simulink model "RC_Servo_Model"  (R2022a)
settings: Solver=VariableStepAuto  StartTime=0.0  StopTime=1  FixedStep=0.001  RelTol=1e-3
undefined symbols (not defined in the file): B, FoV_w, J, K_tau, K_v, La, Pixel_w, Ra
libraries: fl_lib x4, nesl_utility x3, ee_lib x3, simulink_extras x2, simulink x1, slpidlib x1
settings Model: Creator=bobjo  LastModifiedBy=bobjo
settings SolverCC: EnableFixedStepZeroCrossing=on

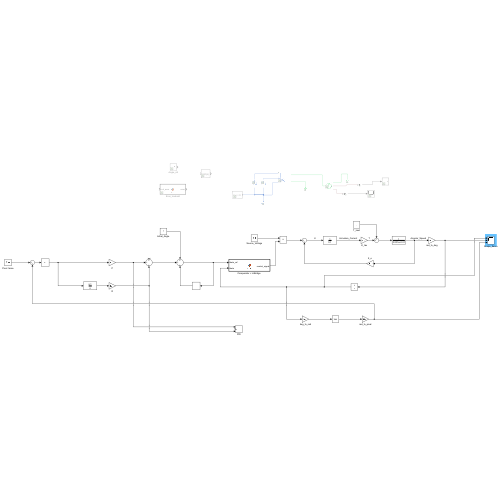
[thumbnail: Simulink's stored preview of the top-level diagram]
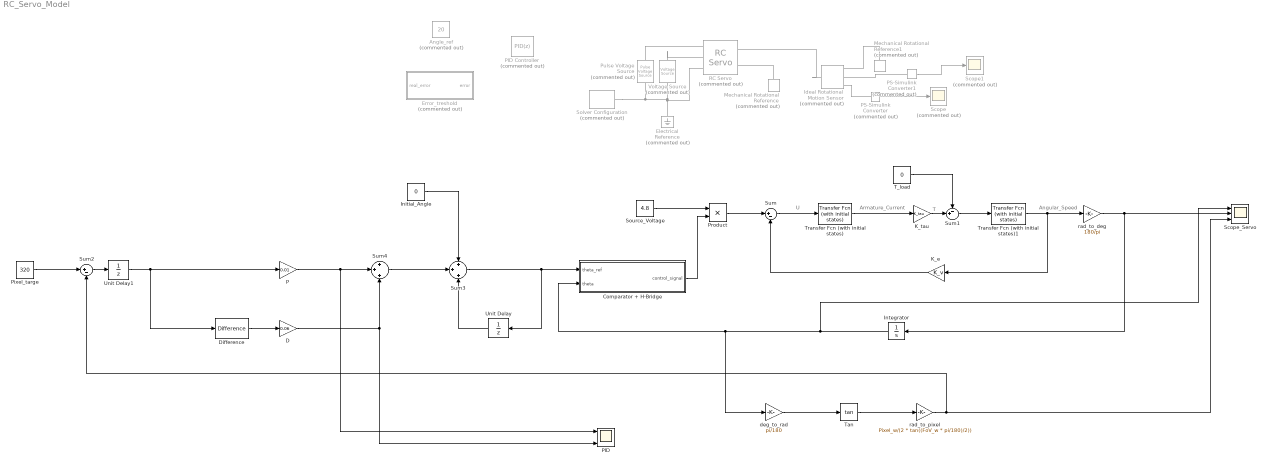
== system RC_Servo_Model ==
  note: Armature_Current
  note: Angular_Speed
  note: T
  note: U
  Angle_ref : Constant  Commented=on  Value=20
  "Comparator + H-Bridge " : MATLAB Function  TreatAsAtomicUnit=on
  D : Gain  Gain=0.06
  Difference : simulink/Discrete/Difference  ICPrevInput=0.0  OutMin=[]  OutMax=[]  OutDataType=fixdt(1, 16)  OutScaling=2^-10  DoSatur=off
  Electrical Reference : fl_lib/Electrical/Electrical Elements/Electrical Reference  Commented=on
      settings: SourceProductBaseCode=PW,SS,VE
  Error_treshold : MATLAB Function  Commented=on  TreatAsAtomicUnit=on
  Ideal Rotational Motion Sensor : fl_lib/Mechanical/Mechanical Sensors/Ideal Rotational Motion Sensor  Commented=on  wrap_angle=simscape.enum.onoff.off  offset=0 rad
      settings: SourceProductBaseCode=PW,SS,VE
  Initial_Angle : Constant  Value=0
  Integrator : Integrator
  K_e : Gain  Gain=K_v
  K_tau : Gain  Gain=K_tau
  Mechanical Rotational Reference : fl_lib/Mechanical/Rotational Elements/Mechanical Rotational Reference  Commented=on
      settings: SourceProductBaseCode=PW,SS,VE
  Mechanical Rotational Reference1 : fl_lib/Mechanical/Rotational Elements/Mechanical Rotational Reference  Commented=on
      settings: SourceProductBaseCode=PW,SS,VE
  P : Gain  Gain=0.01
  PID : Scope  NumInputPorts=3
  PID Controller : slpidlib/PID Controller  Commented=on  Controller=PID  Form=Parallel  TimeDomain=Discrete-time  UseExternalTs=off  SampleTime=0.01  IntegratorMethod=Forward Euler  FilterMethod=Forward Euler  ControllerParametersSource=internal  P=0  I=0  UseKiTs=off  D=0.2 * 0.01  N=100  UseFilter=on  TunerSelectOption=Transfer Function Based (PID Tuner App)  InitialConditionSource=internal  InitialConditionForIntegrator=0  InitialConditionForFilter=0  DifferentiatorICPrevScaledInput=0  ExternalReset=none  TrackingMode=off  Kt=1  LimitOutput=off  SatLimitsSource=internal  UpperSaturationLimit=inf  LowerSaturationLimit=-inf  LinearizeAsGain=on  AntiWindupMode=none  Kb=1  POutMin=[]  POutMax=[]  IOutMin=[]  IOutMax=[]  DOutMin=[]  DOutMax=[]  NOutMin=[]  NOutMax=[]  SumOutMin=[]  SumOutMax=[]  SaturationOutMin=[]  SaturationOutMax=[]  PParamMin=[]  PParamMax=[]  IParamMin=[]  IParamMax=[]  DParamMin=[]  DParamMax=[]  NParamMin=[]  NParamMax=[]  KbParamMin=[]  KbParamMax=[]  KtParamMin=[]  KtParamMax=[]  KbOutMin=[]  KbOutMax=[]  KtOutMin=[]  KtOutMax=[]  IntegratorOutMin=[]  IntegratorOutMax=[]  FilterOutMin=[]  FilterOutMax=[]  SumI1OutMin=[]  SumI1OutMax=[]  SumI2OutMin=[]  SumI2OutMax=[]  SumI3OutMin=[]  SumI3OutMax=[]  SumI4OutMin=[]  SumI4OutMax=[]  SumDOutMin=[]  SumDOutMax=[]  DifferentiatorOutMin=[]  DifferentiatorOutMax=[]  FilterDiffOutCoefMin=[]  FilterDiffOutCoefMax=[]  ReciprocalOutMin=[]  ReciprocalOutMax=[]  SumDenOutMin=[]  SumDenOutMax=[]  SumNumOutMin=[]  SumNumOutMax=[]  DivideOutMin=[]  DivideOutMax=[]  UdiffTsProdOutMin=[]  UdiffTsProdOutMax=[]  NTsProdOutMin=[]  NTsProdOutMax=[]  UintegralTsProdOutMin=[]  UintegralTsProdOutMax=[]  UngainTsProdOutMin=[]  UngainTsProdOutMax=[]  IntegratorContinuousStateAttributes=''  IntegratorStateMustResolveToSignalObject=off  IntegratorRTWStateStorageClass=Auto  FilterContinuousStateAttributes=''  FilterStateMustResolveToSignalObject=off  FilterRTWStateStorageClass=Auto  ParallelPVariant=InternalParameters  IdealPVariant=Disabled  IVariant=InternalParameters  DVariant=InternalParameters  IntegratorVariant=Discrete  SatVariant=Disabled  AWVariant=Passthrough  PCopyVariant=Disabled  TRVariant=Disabled  FdbkBlocksVariant=Forward  IdealPFdbkVariant=Disabled  SatFdbkVariant=Disabled  DerivativeFilterVariant=ForwardEulerFilter  NVariant=InternalParameters  NCopyVariant=Disabled  FilterICVariant=InternalICsFilter  IntegratorICVariant=InternalICs  ExternalResetVariant=Disabled  TRSumVariant=Passthrough  SumFdbkVariant=Disabled  SumVariant=Sum_PID  TsampFilterVariant=InternalTs  TsampNgainVariant=Passthrough  TsampIntegralVariant=Passthrough  ExternalSaturationOutDataTypeStr=Inherit: Same as second input  aMode=0
  PS-Simulink Converter : nesl_utility/PS-Simulink Converter  Commented=on  PhysicalDomain=network_engine_domain  SubClassName=ps_output  LeftPortType=input  RightPortType=output  PseudoPeriodic=off  Frequencies=[]  VectorFormat=inherit  Unit=deg  AffineConversion=off
      settings: SourceProductBaseCode=SS,PW,VE
  PS-Simulink Converter1 : nesl_utility/PS-Simulink Converter  Commented=on  PhysicalDomain=network_engine_domain  SubClassName=ps_output  LeftPortType=input  RightPortType=output  PseudoPeriodic=off  Frequencies=[]  VectorFormat=inherit  Unit=deg/s  AffineConversion=off
      settings: SourceProductBaseCode=SS,PW,VE
  Pixel_targe : Constant  Value=320
  Product : Product
  Pulse Voltage Source : ee_lib/Additional Components/SPICE Sources/Pulse Voltage Source  Commented=on  V1=0 V  V2=5 V  TD=0.1 s  TR=1e-9 s  TF=1e-9 s  PW=0.5 ms  PER=20 ms
      settings: SourceProductBaseCode=PS  InternalSimscapePortConfiguration="{\"Bottom\":[],\"Left\":[{\"id\":\"p\",\"label\":\"\",\"type\":\"foundation.electrical.electrical\"}],\"Right\":[{\"id\":\"n\",\"label\":\"\",\"type\":\"foundation.electrical.electrical\"}],\"Top\":[]}"
  RC Servo : ee_lib/Electromechanical/Brushed Motors/RC Servo  Commented=on  stall_torque=1.8 cm*kg  time_60=0.2 s  nominal_voltage=5 V  rotational_range=[0, 180] deg  pulse_width_range=[500, 2500] us  threshold=3 V  R_s=18 kOhm  resolution=1 deg  angle_meas_error=0 deg  backdrive_torque=0.5 cm*kg  ratio=320  inertia=0.01 cm^2*g  endstop_angles=[-5, 185] deg  endstop_stiffness=1e6 N*m/rad  endstop_damping=0.01 N*m*s/rad  enable_faults=0  fault_action=1  fault_type=1  enable_temporal_fault=0  t_fault=1 s  enable_behavioral_fault=0  max_permissible_current=1 A  t_fail_on_current=1 s  angle_specify=off  angle_priority=High  angle=90 deg  angle_nominal_specify=off  angle_nominal_unit=deg  angle_nominal_value=1  w_specify=off  w_priority=High  w=0 deg/s  w_nominal_specify=off  w_nominal_unit=deg/s  w_nominal_value=1  torque_specify=off  torque_priority=None  torque=0 N*m  torque_nominal_specify=off  torque_nominal_unit=N*m  torque_nominal_value=1  pulse_width_specify=off  pulse_width_priority=Low  pulse_width=1.5 ms  i_specify=off  i_priority=None  i=0 A  i_nominal_specify=off  i_nominal_unit=A  i_nominal_value=1  i_s_specify=off  i_s_priority=None  i_s=0 A  i_s_nominal_specify=off  i_s_nominal_unit=A  i_s_nominal_value=1  motor_torque_specify=off  motor_torque_priority=None  motor_torque=0 N*m  motor_torque_nominal_specify=off  motor_torque_nominal_unit=N*m  motor_torque_nominal_value=1  power_dissipated_specify=off  power_dissipated_priority=None  power_dissipated=0 W  power_dissipated_nominal_specify=off  power_dissipated_nominal_unit=W  power_dissipated_nominal_value=1  angle_demand_specify=off  angle_demand_priority=None  angle_demand=90 deg  angle_demand_nominal_specify=off  angle_demand_nominal_unit=deg  angle_demand_nominal_value=1  faulted_specify=off  faulted_priority=None  faulted=0  faulted_nominal_specify=off  faulted_nominal_unit=1  faulted_nominal_value=1
      settings: SourceProductBaseCode=PS  InternalSimscapePortConfiguration="{\"Bottom\":[],\"Left\":[{\"id\":\"s\",\"label\":\"s\",\"type\":\"foundation.electrical.electrical\"},{\"id\":\"p\",\"label\":\"+\",\"type\":\"foundation.electrical.electrical\"},{\"id\":\"n\",\"label\":\"-\",\"type\":\"foundation.electrical.electrical\"}],\"Right\":[{\"id\":\"R\",\"label\":\"R\",\"type\":\"foundation.mechanical.rotational.rotational\"},{\"id\":\"C\",\"label\":\"C\",\"type\":\"foundation.mechanical.rotational.rotational\"}],\"Top\":[]}"
  Scope : Scope  Commented=on
  Scope1 : Scope  Commented=on
  Scope_Servo : Scope  NumInputPorts=3
  Solver Configuration : nesl_utility/Solver Configuration  Commented=on  PhysicalDomain=network_engine_domain  SubClassName=solver  LeftPortType=input  RightPortType=generic  Tones=[]  Harmonics=[]  SimulateNoise=off  Profile=off  UseLocalSampling=off  EnableSwitchedLinearOptims=on  FrequencyDomain=off  UseCCode=off  RelTol=0.001  AbsTol=0.001  MinStep=1e-09  ToWorkspace=off  RevertToSquareIcSolve=off  NumHomotopyIterations=100  PhasorMode=off  PhasorModeNumHarmonics=1  IndexReductionMethod=DerivativeReplacement  DoDC=off  ResidualTolerance=1e-09  UseLocalSolver=off  LocalSolverChoice=NE_BACKWARD_EULER_ADVANCER  LocalSolverSampleTime=0.001  DoFixedCost=off  MaxNonlinIter=3  MaxModeIter=2  ComputeImpulses=off  ImpulseIterations=2  LinearAlgebra=auto  LinearAlgebraNumThread=0  EquationFormulation=NE_TIME_EF  DelaysMemoryBudget=1024  AutomaticFiltering=on  FilteringTimeConstant=0.001  PartitionStorageMethod=AS_NEEDED  PartitionMemoryBudget=1024  PartitionMethod=ROBUST
      settings: SourceProductBaseCode=SS,PW,VE
  Source_Voltage : Constant  Value=4.8
  Sum : Sum  Inputs=|+-
  Sum1 : Sum  Inputs=-+|
  Sum2 : Sum  Inputs=|+-
  Sum3 : Sum  Inputs=+|+|+
  Sum4 : Sum  Inputs=+|+|+
  T_load : Constant  Value=0
  Tan : Trigonometry  Operator=tan
  Transfer Fcn (with initial states) : simulink_extras/Additional Linear/Transfer Fcn (with initial states)  N=[1]  D="[La  Ra]"  X0=0
  Transfer Fcn (with initial states)1 : simulink_extras/Additional Linear/Transfer Fcn (with initial states)  N=[1]  D="[J  B]"  X0=0
  Unit Delay : UnitDelay  SampleTime=0.01  HasFrameUpgradeWarning=on
  Unit Delay1 : UnitDelay  SampleTime=0.01  HasFrameUpgradeWarning=on
  Voltage Source : ee_lib/Sources/Voltage Source  Commented=on  dc_voltage=5 V  ac_voltage=0 V  ac_shift=0 rad  ac_frequency=0 Hz  noise_mode=0  PSD=0 V^2/Hz  repeatability=1  auto_seed=3499211588  user_seed=0  sample_time=1e-3 s  i_specify=off  i_priority=None  i=0 A  i_nominal_specify=off  i_nominal_unit=A  i_nominal_value=1  v_specify=off  v_priority=None  v=0 V  v_nominal_specify=off  v_nominal_unit=V  v_nominal_value=1
  deg_to_rad : Gain  Gain=pi/180
  rad_to_deg : Gain  Gain=180/pi
  rad_to_pixel : Gain  Gain=Pixel_w/(2 * tan((FoV_w * pi/180)/2))
  wires:
  PS-Simulink Converter/1 -> Scope/1
  Sum/1 -> Transfer Fcn (with initial states)/1
  Transfer Fcn (with initial states)/1 -> K_tau/1
  T_load/1 -> Sum1/1
  K_tau/1 -> Sum1/2
  Sum1/1 -> Transfer Fcn (with initial states)1/1
  K_e/1 -> Sum/2
  rad_to_deg/1 -> Scope_Servo/2, Integrator/1
  PS-Simulink Converter1/1 -> Scope1/1
  Product/1 -> Sum/1
  Source_Voltage/1 -> Product/1
  Transfer Fcn (with initial states)1/1 -> K_e/1, rad_to_deg/1
  Tan/1 -> rad_to_pixel/1
  deg_to_rad/1 -> Tan/1
  Pixel_targe/1 -> Sum2/1
  Integrator/1 -> deg_to_rad/1, "Comparator + H-Bridge "/2(theta), Scope_Servo/1
  "Comparator + H-Bridge "/1(control_signal) -> Product/2
  Sum3/1 -> Unit Delay/1, "Comparator + H-Bridge "/1(theta_ref)
  Unit Delay/1 -> Sum3/3
  Initial_Angle/1 -> Sum3/1
  P/1 -> Sum4/2, PID/1
  Sum4/1 -> Sum3/2
  Difference/1 -> D/1
  D/1 -> PID/3, Sum4/3
  rad_to_pixel/1 -> Sum2/2, Scope_Servo/3
  Sum2/1 -> Unit Delay1/1
  Unit Delay1/1 -> Difference/1, P/1
  connections:
  Pulse Voltage Source/LConn1 -- RC Servo/LConn1
  Pulse Voltage Source/RConn1 -- Solver Configuration/RConn1 -- Electrical Reference/LConn1 -- RC Servo/LConn3 -- Voltage Source/RConn1
  Voltage Source/LConn1 -- RC Servo/LConn2
  Mechanical Rotational Reference/LConn1 -- RC Servo/RConn2
  Ideal Rotational Motion Sensor/LConn1 -- RC Servo/RConn1
  Ideal Rotational Motion Sensor/RConn3 -- PS-Simulink Converter/LConn1
  Mechanical Rotational Reference1/LConn1 -- Ideal Rotational Motion Sensor/RConn1
  PS-Simulink Converter1/LConn1 -- Ideal Rotational Motion Sensor/RConn2

== matlab function RC_Servo_Model/Comparator + H-Bridge  ==
  data: theta_ref input; control_signal output; theta input
function control_signal = comp(theta_ref, theta)

control_signal = 0;

if(theta_ref < theta)
    control_signal = -1;
end

if(theta_ref > theta)
    control_signal = 1;
end

if(abs(theta_ref - theta) < 1)
    control_signal = 0;
end

== matlab function RC_Servo_Model/Error_treshold ==
  data: real_error input; error output
function  error = fcn(real_error)

error = real_error;

if(abs(real_error) < 16)
    error = 0;
end
